simulink model "GEO_insertion"  (R2023b)
settings: Solver=FixedStepAuto  StartTime=0.0  StopTime=60*60*24*20  FixedStep=60  RelTol=1e-3
values from neighbouring files (symbols this model uses):
  A = 42164500    [GEO_insertion_setup.m]
  ext_ENV_muEarth = 3.986005e14    (= 398600500000000)    [GEO_insertion_setup.m]    (also in HSat_op_setup.m; HSat_op_setup_merged_maria.m; init_orbit_analysis_with_drag_loss.m)
  lambda_GEO = 79*pi/180    (= 1.37881010908)    [GEO_insertion_setup.m]
  OR_thrusterforce = 50e-3    (= 0.05)    [GEO_insertion_setup.m]    (also in HSat_op_setup.m = 0.275; HSat_op_setup_merged_maria.m = 0.275)
  psi_rads = 7.2921e-05    [GEO_insertion_setup.m]
  SC_mass = 500    [GEO_insertion_setup.m]
  sim_start = juliandate(2020, 1, 1, 12, 0, 0)    [GEO_insertion_setup.m]    (also in HSat_op_setup.m = ymd2jd(YYYY,MM,DD,'gregorian')-.5+hh/24+mm/1440+ss/86400; HSat_op_setup_merged_maria.m = ymd2jd(YYYY,MM,DD,'gregorian')-.5+hh/24+mm/1440+ss/86400)
  thrust_acc = OR_thrusterforce/SC_mass    (= 0.0001)    [GEO_insertion_setup.m]
undefined symbols (not defined in the file or in its folder): pos_start, vel_start
libraries: simulink x4, aerolibutil x2, sharedtransform x1, matrix_library x1
(part 2 of 2)

== system GEO_insertion/Subsystem/Subsystem2/Subsystem7/Subsystem5/Subsystem ==
  nu : Inport
  eabs : Inport  Port=2
  Constant1 : Constant
  Constant2 : Constant  Value=2*pi
  Divide1 : Product  Inputs=**
  Math Function : Math  Operator=square
  Math Function1 : Math  Operator=mod
  Sqrt : Sqrt
  Sum1 : Sum  Inputs=|+-
  Sum3 : Sum  Inputs=|++
  Trigonometric Function1 : Trigonometry  Operator=atan2
  Trigonometric Function2 : Trigonometry  Operator=cos
  Trigonometric Function3 : Trigonometry
  E : Outport
  wires:
  eabs/1 -> Math Function/1, Sum3/1
  nu/1 -> Trigonometric Function3/1, Trigonometric Function2/1
  Trigonometric Function2/1 -> Sum3/2
  Sum3/1 -> Trigonometric Function1/2
  Trigonometric Function1/1 -> Math Function1/1
  Sum1/1 -> Sqrt/1
  Math Function/1 -> Sum1/2
  Constant1/1 -> Sum1/1
  Sqrt/1 -> Divide1/1
  Trigonometric Function3/1 -> Divide1/2
  Divide1/1 -> Trigonometric Function1/1
  Math Function1/1 -> E/1
  Constant2/1 -> Math Function1/2

== system GEO_insertion/Subsystem/Subsystem2/Subsystem7/Subsystem5/Subsystem1 ==
  E : Inport
  eabs : Inport  Port=2
  Constant2 : Constant  Value=2*pi
  Divide1 : Product  Inputs=**
  Math Function1 : Math  Operator=mod
  Sum : Sum  Inputs=|+-
  Trigonometric Function1 : Trigonometry
  M : Outport
  wires:
  Sum/1 -> Math Function1/1  "M"
  eabs/1 -> Divide1/2
  E/1 -> Sum/1, Trigonometric Function1/1
  Divide1/1 -> Sum/2  "e"
  Trigonometric Function1/1 -> Divide1/1
  Constant2/1 -> Math Function1/2
  Math Function1/1 -> M/1

== system GEO_insertion/Subsystem/Subsystem2/Subsystem7/Subsystem5/Subsystem2 ==
  e : Inport
  r : Inport  Port=2
  eabs : Inport  Port=3
  rabs : Inport  Port=4
  Divide8 : Product  Inputs=*/
  Divide9 : Product  Inputs=**
  Dot Product1 : DotProduct  OutDataTypeStr=Inherit: Inherit via internal rule
  Trigonometric Function2 : Trigonometry  Operator=acos
  nu : Outport
  wires:
  eabs/1 -> Divide9/1
  Trigonometric Function2/1 -> nu/1  "nu"
  r/1 -> Dot Product1/2
  rabs/1 -> Divide9/2
  Divide8/1 -> Trigonometric Function2/1
  e/1 -> Dot Product1/1
  Divide9/1 -> Divide8/2  "e"
  Dot Product1/1 -> Divide8/1

== system GEO_insertion/Subsystem/Subsystem2/Subsystem7/Subsystem5/Subsystem3 ==
  E : Inport
  eabs : Inport  Port=2
  Constant : Constant
  Constant1 : Constant
  Divide2 : Product  Inputs=**
  Divide3 : Product  Inputs=*/
  Gain : Gain  Gain=2
  Gain1 : Gain  Gain=.5
  Sqrt : Sqrt
  Sum1 : Sum  Inputs=|++
  Sum2 : Sum  Inputs=|+-
  Trigonometric Function3 : Trigonometry  Operator=atan
  Trigonometric Function4 : Trigonometry  Operator=tan
  nu : Outport
  wires:
  Sqrt/1 -> Divide2/2
  Gain1/1 -> Trigonometric Function4/1
  Constant1/1 -> Sum2/1
  Sum2/1 -> Divide3/2
  eabs/1 -> Sum2/2, Sum1/2
  E/1 -> Gain1/1
  Sum1/1 -> Divide3/1
  Trigonometric Function3/1 -> Gain/1
  Trigonometric Function4/1 -> Divide2/1
  Divide2/1 -> Trigonometric Function3/1
  Constant/1 -> Sum1/1
  Divide3/1 -> Sqrt/1
  Gain/1 -> nu/1  "E"

== system GEO_insertion/Subsystem1/Switch Case Action Subsystem2/Switch Case Action Subsystem/Subsystem1/go to D = 0 ==
  D : Inport
  Constant : Constant  Value=A
  Constant1 : Constant  Value=psi_rads
  Constant2 : Constant  Value=-3*361
  Constant3 : Constant  Value=thrust_acc
  Divide : Product  Inputs=***/
  Divide1 : Product  Inputs=*/
  Divide2 : Product  Inputs=*/
  Gain : Gain  Gain=1/2
  dV (m/s) : Outport
  thrust_time (s) : Outport  Port=2
  dlambda_start : Outport  Port=3
  wires:
  D/1 -> Divide2/1, Divide/1
  Constant/1 -> Divide/2
  Constant1/1 -> Divide/3
  Constant2/1 -> Divide/4
  Divide/1 -> Divide1/1, dV (m/s)/1
  Constant3/1 -> Divide1/2
  Divide1/1 -> Gain/1, thrust_time (s)/1
  Gain/1 -> Divide2/2
  Divide2/1 -> dlambda_start/1

== system GEO_insertion/Subsystem1/Switch Case Action Subsystem2/Switch Case Action Subsystem1/Subsystem1/go to D = 0 ==
  D : Inport
  Constant : Constant  Value=A
  Constant1 : Constant  Value=psi_rads
  Constant2 : Constant  Value=-3*361
  Constant3 : Constant  Value=thrust_acc
  Divide : Product  Inputs=***/
  Divide1 : Product  Inputs=*/
  Divide2 : Product  Inputs=*/
  Gain : Gain  Gain=1/2
  dV (m/s) : Outport
  thrust_time (s) : Outport  Port=2
  dlambda_start : Outport  Port=3
  wires:
  D/1 -> Divide2/1, Divide/1
  Constant/1 -> Divide/2
  Constant1/1 -> Divide/3
  Constant2/1 -> Divide/4
  Divide/1 -> Divide1/1, dV (m/s)/1
  Constant3/1 -> Divide1/2
  Divide1/1 -> Gain/1, thrust_time (s)/1
  Gain/1 -> Divide2/2
  Divide2/1 -> dlambda_start/1

== matlab function GEO_insertion/Subsystem/Subsystem/MATLAB Function ==
  data: r input; coe output; v input
%SV2KEP.M
%
%function kepvec=sv2kep(rsc,vsc)
%
%DESCRIPTION
%Converts from state vector (rvec,vvec) formulation to keplerian elements
%
%INPUT:		rsc	 (3x1) or (3xn) orbit radius vector
%				vsc (3x1) or (3xn) velocity vector
%
%OUTPUT:    	kepvec - (6x1) or (6xn) vector with the keplerian elements
%USES:
%REFERENCE:
%AUTHOR:      	B Jakobsson
%VERSION: 	   92-08-17
%	   	      95-10-02
%				BJA, Sept 2001, vector input accepted, vector output added

% function coe=sv2kep(rvec,vvec)
% 
% if 0
% [p,sma,ecc,incl,an,ap,tran,E,M,arglat,truelon,lonper ] = rv2coe (rvec,vvec);
% coe=[sma ecc incl an ap tran, E, M,arglat,truelon,lonper ]';
% else
%     coe = rv2coe (rvec,vvec);
% end
  
%
% ------------------------------------------------------------------------------
%
%                           function rv2coe
%
%  this function finds the classical orbital elements given the geocentric
%    equatorial position and velocity vectors.
%
%  author        : david vallado                  719-573-2600   21 jun 2002
%
%  revisions
%    vallado     - fix special cases                              5 sep 2002
%    vallado     - delete extra check in inclination code        16 oct 2002
%    vallado     - add constant file use                         29 jun 2003
%    vallado     - add mu                                         2 apr 2007
%
%  inputs          description                    range / units
%    r           - ijk position vector            km
%    v           - ijk velocity vector            km / s
%    mu          - gravitational parameter        km3 / s2
%
%  outputs       :
%    p           - semilatus rectum               km
%    a           - semimajor axis                 km
%    ecc         - eccentricity
%    incl        - inclination                    0.0  to pi rad
%    omega       - longitude of ascending node    0.0  to 2pi rad
%    argp        - argument of perigee            0.0  to 2pi rad
%    nu          - true anomaly                   0.0  to 2pi rad
%    m           - mean anomaly                   0.0  to 2pi rad
%    arglat      - argument of latitude      (ci) 0.0  to 2pi rad
%    truelon     - true longitude            (ce) 0.0  to 2pi rad
%    lonper      - longitude of periapsis    (ee) 0.0  to 2pi rad
%
%  locals        :
%    hbar        - angular momentum h vector      km2 / s
%    ebar        - eccentricity     e vector
%    nbar        - line of nodes    n vector
%    c1          - v**2 - u/r
%    rdotv       - r dot v
%    hk          - hk unit vector
%    sme         - specfic mechanical energy      km2 / s2
%    i           - index
%    e           - eccentric, parabolic,
%                  hyperbolic anomaly             rad
%    temp        - temporary variable
%    typeorbit   - type of orbit                  ee, ei, ce, ci
%
%  coupling      :
%    mag         - magnitude of a vector
%    angl        - find the angl between two vectors
%    newtonnu    - find the mean anomaly
%
%  references    :
%    vallado       2007, 121, alg 9, ex 2-5
%
% [p,a,ecc,incl,omega,argp,nu,m,arglat,truelon,lonper ] = rv2coe (r,v);
% ------------------------------------------------------------------------------

  %  function [p,a,ecc,incl,omega,argp,nu,e,m,arglat,truelon,lonper ] = rv2coe (r,v);
     function coe = rv2coe (r,v)
        
        %  constmath;
        small=1e-10;
        infinite  = 999999.9;
        undefined = 999999.1;
        % -------------------------  mathematical  --------------------
        rad    = 180.0 / pi;
        twopi  = 2.0 * pi;
        halfpi = pi * 0.5;
        
        % constastro;  % don't overwrite mu
        mu=3.986005e14;
        muin = mu; % this is the km version
        % -------------------------  implementation   -----------------
        magr = norm( r );
        magv = norm( v );
        % ------------------  find h n and e vectors   ----------------
        [hbar] = cross( r,v );
        nbar=hbar*NaN;
        ebar=hbar*NaN;
        magh = mag( hbar );
        if ( magh > small )
            nbar(1)= -hbar(2);
            nbar(2)=  hbar(1);
            nbar(3)=   0.0;
            magn = mag( nbar );
            c1 = magv*magv - muin /magr;
            rdotv= dot( r,v );
            for i= 1 : 3
                ebar(i)= (c1*r(i) - rdotv*v(i))/muin;
            end
            ecc = mag( ebar );
            
            % ------------  find a e and semi-latus rectum   ----------
            sme= ( magv*magv*0.5  ) - ( muin /magr );
            if ( abs( sme ) > small )
                a= -muin  / (2.0 *sme);
            else
                a= infinite;
            end
            p = magh*magh/muin;
            
            % -----------------  find inclination   -------------------
            hk= hbar(3)/magh;
            incl= acos( hk );
            
            % --------  determine type of orbit for later use  --------
            % ------ elliptical, parabolic, hyperbolic inclined -------
            typeorbit= 'ei';
            if ( ecc < small )
                % ----------------  circular equatorial ---------------
                if  (incl<small) || (abs(incl-pi)<small)
                    typeorbit= 'ce';
                else
                    % --------------  circular inclined ---------------
                    typeorbit= 'ci';
                end
            else
                % - elliptical, parabolic, hyperbolic equatorial --
                if  (incl<small) || (abs(incl-pi)<small)
                    typeorbit= 'ee';
                end
            end
            
            % ----------  find longitude of ascending node ------------
            if ( magn > small )
                temp= nbar(1) / magn;
                if ( abs(temp) > 1.0  )
                    temp= sign(temp);
                end
                omega= acos( temp );
                if ( nbar(2) < 0.0  )
                    omega= twopi - omega;
                end
            else
                omega= undefined;
            end
            
            % ---------------- find argument of perigee ---------------
            if (strcmp(typeorbit, 'ei') == 1)
                argp = angl( nbar,ebar);
                if ( ebar(3) < 0.0  )
                    argp= twopi - argp;
                end
            else
                argp= undefined;
            end
            
            % ------------  find true anomaly at epoch    -------------
            if ( typeorbit(1:1) == 'e' )
                nu =  angl( ebar,r);
                if ( rdotv < 0.0  )
                    nu= twopi - nu;
                end
            else
                nu= undefined;
            end
            
            % ----  find argument of latitude - circular inclined -----
            if (strcmp(typeorbit, 'ci') == 1)
                arglat = angl( nbar,r );
                if ( r(3) < 0.0  )
                    arglat= twopi - arglat;
                end
                m = arglat;
            else
                arglat= undefined;
            end
            
            % -- find longitude of perigee - elliptical equatorial ----
            if  ( ecc>small ) && (strcmp(typeorbit, 'ee') == 1)
                temp= ebar(1)/ecc;
                if ( abs(temp) > 1.0  )
                    temp= sign(temp);
                end
                lonper= acos( temp );
                if ( ebar(2) < 0.0  )
                    lonper= twopi - lonper;
                end
                if ( incl > halfpi )
                    lonper= twopi - lonper;
                end
            else
                lonper= undefined;
            end
            
            % -------- find true longitude - circular equatorial ------
            if  ( magr>small ) && (strcmp(typeorbit, 'ce') == 1)
                temp= r(1)/magr;
                if ( abs(temp) > 1.0  )
                    temp= sign(temp);
                end
                truelon= acos( temp );
                if ( r(2) < 0.0  )
                    truelon= twopi - truelon;
                end
                if ( incl > halfpi )
                    truelon= twopi - truelon;
                end
                m = truelon;
            else
                truelon= undefined;
            end
            
            % ------------ find mean anomaly for all orbits -----------
            if ( typeorbit(1:1) == 'e' )
                [e,m] = newtonnu(ecc,nu );
            else
                e=undefined;
                m=undefined;
                
            end
            
        else
            p    = undefined;
            a    = undefined;
            ecc  = undefined;
            incl = undefined;
            omega= undefined;
            argp = undefined;
            nu   = undefined;
            m    = undefined;
            e    = undefined;
            arglat = undefined;
            truelon= undefined;
            lonper = undefined;
        end
%coe=[sma ecc incl an ap tran, E, M,arglat,truelon,lonper ]
coe=[  a,ecc,incl,omega,argp,nu,e,m,arglat,truelon,lonper ]';
    end
% end

== matlab function GEO_insertion/Subsystem/Subsystem2/Subsystem1/MATLAB Function ==
  data: jd input; G output
function G = getG(jd)

[year_jd,psi]=getG0relation;
G0=interp1(year_jd,psi,jd,'previous','extrap');
year0_jd_idx=find(psi==G0,1);
year0_jd=year_jd(year0_jd_idx(1));

ddoy=jd-year0_jd;

G=(G0+360.985647*ddoy)*pi/180;

function [year_jd,psi]=getG0relation
%year	G	days/year
M=[  2444240 1980  99.814 366
     2444606 1981 100.561 365
     2444971 1982 100.322 365
     2445336 1983 100.083 365
     2445701 1984  99.845 366
     2446067 1985 100.592 365
     2446432 1986 100.353 365
     2446797 1987 100.114 365
     2447162 1988  99.875 366
     2447528 1989 100.622 365
     2447893 1990 100.384 365
     2448258 1991 100.145 365
     2448623 1992  99.906 366
     2448989 1993 100.653 365
     2449354 1994 100.414 365
     2449719 1995 100.176 365
     2450084 1996  99.937 366
     2450450 1997 100.684 365
     2450815 1998 100.445 365
     2451180 1999 100.207 365
     2451545 2000  99.968 366
     2451911 2001 100.715 365
     2452276 2002 100.476 365
     2452641 2003 100.237 365
     2453006 2004  99.999 366
     2453372 2005 100.746 365
     2453737 2006 100.507 365
     2454102 2007 100.268 365
     2454467 2008 100.029 366
     2454833 2009 100.776 365
     2455198 2010 100.538 365
     2455563 2011 100.299 365
     2455928 2012 100.060 366
     2456294 2013 100.807 365
     2456659 2014 100.568 365
     2457024 2015 100.330 365
     2457389 2016 100.091 366
     2457755 2017 100.838 365
     2458120 2018 100.599 365
     2458485 2019 100.361 365
     2458850 2020 100.122 366
     2459216 2021 100.869 365
     2459581 2022 100.630 365
     2459946 2023 100.391 365
     2460311 2024 100.153 366
     2460677 2025 100.900 365
     2461042 2026 100.661 365
     2461407 2027 100.422 365
     2461772 2028 100.183 366
     2462138 2029 100.930 365
     2462503 2030 100.692 365
     2462868 2031 100.453 365
     2463233 2032 100.214 366
     2463599 2033 100.961 365
     2463964 2034 100.722 365
     2464329 2035 100.484 365
     2464694 2036 100.245 366
     2465060 2037 100.992 365
     2465425 2038 100.753 365
     2465790 2039 100.515 365
     2466155 2040 100.276 366
     2466521 2041 101.023 365
     2466886 2042 100.784 365
     2467251 2043 100.545 365];
year_jd=M(:,1);
psi=M(:,3);
end



end
